simulink model "PID_Controller_Quadrotor"  (R2019b)
settings: Solver=VariableStepAuto  StartTime=0.0  StopTime=200  RelTol=1e-3
values from neighbouring files (symbols this model uses):
  b = 6.66e-5    (= 6.66e-05)    [LQR control.m]    (also in Parameters for PID.m)
  d = 1.642e-4    (= 0.0001642)    [Parameters for PID.m]
  g = 9.81    [Parameters for PID.m]
  Ixx = 155237782e-9    (= 0.155237782)    [LQR control.m]    (also in Parameters for PID.m)
  Iyy = 183039510e-9    (= 0.18303951)    [LQR control.m]    (also in Parameters for PID.m)
  Izz = 66119823e-9    (= 0.066119823)    [LQR control.m]    (also in Parameters for PID.m)
  Jr = 824e-6    (= 0.000824)    [Parameters for PID.m]
  l = 0.34    [Parameters for PID.m]
  m = 4    [LQR control.m]    (also in Parameters for PID.m)
undefined symbols (not defined in the file or in its folder): sigbuilder_block
libraries: simulink x4
settings Model: Creator=Dell  LastModifiedBy=Dell

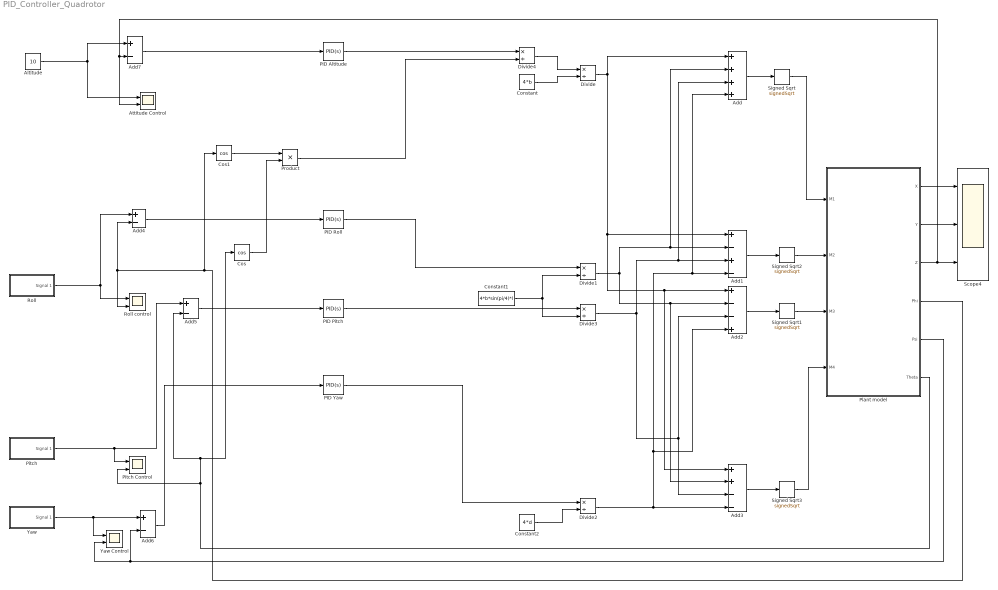
== system PID_Controller_Quadrotor ==
  " PID Altitude" : simulink/Continuous/PID Controller  Controller=PID  Form=Parallel  TimeDomain=Continuous-time  SampleTime=-1  IntegratorMethod=Forward Euler  FilterMethod=Forward Euler  ControllerParametersSource=internal  P=10  I=1.5  D=4.7  UseFilter=on  N=100  TunerSelectOption=Transfer Function Based (PID Tuner App)  InitialConditionSource=internal  InitialConditionForIntegrator=0  InitialConditionForFilter=0  DifferentiatorICPrevScaledInput=0  ExternalReset=none  TrackingMode=off  Kt=1  LimitOutput=off  UpperSaturationLimit=inf  LowerSaturationLimit=-inf  LinearizeAsGain=off  AntiWindupMode=none  Kb=1  POutMin=[]  POutMax=[]  IOutMin=[]  IOutMax=[]  DOutMin=[]  DOutMax=[]  NOutMin=[]  NOutMax=[]  SumOutMin=[]  SumOutMax=[]  SaturationOutMin=[]  SaturationOutMax=[]  PParamMin=[]  PParamMax=[]  IParamMin=[]  IParamMax=[]  DParamMin=[]  DParamMax=[]  NParamMin=[]  NParamMax=[]  KbParamMin=[]  KbParamMax=[]  KtParamMin=[]  KtParamMax=[]  KbOutMin=[]  KbOutMax=[]  KtOutMin=[]  KtOutMax=[]  IntegratorOutMin=[]  IntegratorOutMax=[]  FilterOutMin=[]  FilterOutMax=[]  SumI1OutMin=[]  SumI1OutMax=[]  SumI2OutMin=[]  SumI2OutMax=[]  SumI3OutMin=[]  SumI3OutMax=[]  SumI4OutMin=[]  SumI4OutMax=[]  SumDOutMin=[]  SumDOutMax=[]  DifferentiatorOutMin=[]  DifferentiatorOutMax=[]  FilterDiffOutCoefMin=[]  FilterDiffOutCoefMax=[]  ReciprocalOutMin=[]  ReciprocalOutMax=[]  SumDenOutMin=[]  SumDenOutMax=[]  SumNumOutMin=[]  SumNumOutMax=[]  DivideOutMin=[]  DivideOutMax=[]  IntegratorContinuousStateAttributes=''  IntegratorStateMustResolveToSignalObject=off  IntegratorRTWStateStorageClass=Auto  FilterContinuousStateAttributes=''  FilterStateMustResolveToSignalObject=off  FilterRTWStateStorageClass=Auto  ParallelPVariant=InternalParameters  IdealPVariant=Disabled  IVariant=InternalParameters  DVariant=InternalParameters  IntegratorVariant=Continuous  SatVariant=Disabled  AWVariant=Passthrough  PCopyVariant=Disabled  TRVariant=Disabled  FdbkBlocksVariant=Forward  IdealPFdbkVariant=Disabled  SatFdbkVariant=Disabled  DerivativeFilterVariant=ContFilter  NVariant=InternalParameters  NCopyVariant=Disabled  FilterICVariant=InternalICsFilter  IntegratorICVariant=InternalICs  ExternalResetVariant=Disabled  TRSumVariant=Passthrough  SumFdbkVariant=Disabled  SumVariant=Sum_PID
  " PID Pitch" : simulink/Continuous/PID Controller  Controller=PID  Form=Parallel  TimeDomain=Continuous-time  SampleTime=-1  IntegratorMethod=Forward Euler  FilterMethod=Forward Euler  ControllerParametersSource=internal  P=0.04  I=0  D=0.6  UseFilter=on  N=100  TunerSelectOption=Transfer Function Based (PID Tuner App)  InitialConditionSource=internal  InitialConditionForIntegrator=0  InitialConditionForFilter=0  DifferentiatorICPrevScaledInput=0  ExternalReset=none  TrackingMode=off  Kt=1  LimitOutput=off  UpperSaturationLimit=inf  LowerSaturationLimit=-inf  LinearizeAsGain=off  AntiWindupMode=none  Kb=1  POutMin=[]  POutMax=[]  IOutMin=[]  IOutMax=[]  DOutMin=[]  DOutMax=[]  NOutMin=[]  NOutMax=[]  SumOutMin=[]  SumOutMax=[]  SaturationOutMin=[]  SaturationOutMax=[]  PParamMin=[]  PParamMax=[]  IParamMin=[]  IParamMax=[]  DParamMin=[]  DParamMax=[]  NParamMin=[]  NParamMax=[]  KbParamMin=[]  KbParamMax=[]  KtParamMin=[]  KtParamMax=[]  KbOutMin=[]  KbOutMax=[]  KtOutMin=[]  KtOutMax=[]  IntegratorOutMin=[]  IntegratorOutMax=[]  FilterOutMin=[]  FilterOutMax=[]  SumI1OutMin=[]  SumI1OutMax=[]  SumI2OutMin=[]  SumI2OutMax=[]  SumI3OutMin=[]  SumI3OutMax=[]  SumI4OutMin=[]  SumI4OutMax=[]  SumDOutMin=[]  SumDOutMax=[]  DifferentiatorOutMin=[]  DifferentiatorOutMax=[]  FilterDiffOutCoefMin=[]  FilterDiffOutCoefMax=[]  ReciprocalOutMin=[]  ReciprocalOutMax=[]  SumDenOutMin=[]  SumDenOutMax=[]  SumNumOutMin=[]  SumNumOutMax=[]  DivideOutMin=[]  DivideOutMax=[]  IntegratorContinuousStateAttributes=''  IntegratorStateMustResolveToSignalObject=off  IntegratorRTWStateStorageClass=Auto  FilterContinuousStateAttributes=''  FilterStateMustResolveToSignalObject=off  FilterRTWStateStorageClass=Auto  ParallelPVariant=InternalParameters  IdealPVariant=Disabled  IVariant=InternalParameters  DVariant=InternalParameters  IntegratorVariant=Continuous  SatVariant=Disabled  AWVariant=Passthrough  PCopyVariant=Disabled  TRVariant=Disabled  FdbkBlocksVariant=Forward  IdealPFdbkVariant=Disabled  SatFdbkVariant=Disabled  DerivativeFilterVariant=ContFilter  NVariant=InternalParameters  NCopyVariant=Disabled  FilterICVariant=InternalICsFilter  IntegratorICVariant=InternalICs  ExternalResetVariant=Disabled  TRSumVariant=Passthrough  SumFdbkVariant=Disabled  SumVariant=Sum_PID
  " PID Roll" : simulink/Continuous/PID Controller  Controller=PID  Form=Parallel  TimeDomain=Continuous-time  SampleTime=-1  IntegratorMethod=Forward Euler  FilterMethod=Forward Euler  ControllerParametersSource=internal  P=0.001  I=0  D=0.13  UseFilter=on  N=100  TunerSelectOption=Transfer Function Based (PID Tuner App)  InitialConditionSource=internal  InitialConditionForIntegrator=0  InitialConditionForFilter=0  DifferentiatorICPrevScaledInput=0  ExternalReset=none  TrackingMode=off  Kt=1  LimitOutput=off  UpperSaturationLimit=inf  LowerSaturationLimit=-inf  LinearizeAsGain=off  AntiWindupMode=none  Kb=1  POutMin=[]  POutMax=[]  IOutMin=[]  IOutMax=[]  DOutMin=[]  DOutMax=[]  NOutMin=[]  NOutMax=[]  SumOutMin=[]  SumOutMax=[]  SaturationOutMin=[]  SaturationOutMax=[]  PParamMin=[]  PParamMax=[]  IParamMin=[]  IParamMax=[]  DParamMin=[]  DParamMax=[]  NParamMin=[]  NParamMax=[]  KbParamMin=[]  KbParamMax=[]  KtParamMin=[]  KtParamMax=[]  KbOutMin=[]  KbOutMax=[]  KtOutMin=[]  KtOutMax=[]  IntegratorOutMin=[]  IntegratorOutMax=[]  FilterOutMin=[]  FilterOutMax=[]  SumI1OutMin=[]  SumI1OutMax=[]  SumI2OutMin=[]  SumI2OutMax=[]  SumI3OutMin=[]  SumI3OutMax=[]  SumI4OutMin=[]  SumI4OutMax=[]  SumDOutMin=[]  SumDOutMax=[]  DifferentiatorOutMin=[]  DifferentiatorOutMax=[]  FilterDiffOutCoefMin=[]  FilterDiffOutCoefMax=[]  ReciprocalOutMin=[]  ReciprocalOutMax=[]  SumDenOutMin=[]  SumDenOutMax=[]  SumNumOutMin=[]  SumNumOutMax=[]  DivideOutMin=[]  DivideOutMax=[]  IntegratorContinuousStateAttributes=''  IntegratorStateMustResolveToSignalObject=off  IntegratorRTWStateStorageClass=Auto  FilterContinuousStateAttributes=''  FilterStateMustResolveToSignalObject=off  FilterRTWStateStorageClass=Auto  ParallelPVariant=InternalParameters  IdealPVariant=Disabled  IVariant=InternalParameters  DVariant=InternalParameters  IntegratorVariant=Continuous  SatVariant=Disabled  AWVariant=Passthrough  PCopyVariant=Disabled  TRVariant=Disabled  FdbkBlocksVariant=Forward  IdealPFdbkVariant=Disabled  SatFdbkVariant=Disabled  DerivativeFilterVariant=ContFilter  NVariant=InternalParameters  NCopyVariant=Disabled  FilterICVariant=InternalICsFilter  IntegratorICVariant=InternalICs  ExternalResetVariant=Disabled  TRSumVariant=Passthrough  SumFdbkVariant=Disabled  SumVariant=Sum_PID
  " PID Yaw" : simulink/Continuous/PID Controller  Controller=PID  Form=Parallel  TimeDomain=Continuous-time  SampleTime=-1  IntegratorMethod=Forward Euler  FilterMethod=Forward Euler  ControllerParametersSource=internal  P=0.001  I=0  D=0.6  UseFilter=on  N=100  TunerSelectOption=Transfer Function Based (PID Tuner App)  InitialConditionSource=internal  InitialConditionForIntegrator=0  InitialConditionForFilter=0  DifferentiatorICPrevScaledInput=0  ExternalReset=none  TrackingMode=off  Kt=1  LimitOutput=off  UpperSaturationLimit=inf  LowerSaturationLimit=-inf  LinearizeAsGain=off  AntiWindupMode=none  Kb=1  POutMin=[]  POutMax=[]  IOutMin=[]  IOutMax=[]  DOutMin=[]  DOutMax=[]  NOutMin=[]  NOutMax=[]  SumOutMin=[]  SumOutMax=[]  SaturationOutMin=[]  SaturationOutMax=[]  PParamMin=[]  PParamMax=[]  IParamMin=[]  IParamMax=[]  DParamMin=[]  DParamMax=[]  NParamMin=[]  NParamMax=[]  KbParamMin=[]  KbParamMax=[]  KtParamMin=[]  KtParamMax=[]  KbOutMin=[]  KbOutMax=[]  KtOutMin=[]  KtOutMax=[]  IntegratorOutMin=[]  IntegratorOutMax=[]  FilterOutMin=[]  FilterOutMax=[]  SumI1OutMin=[]  SumI1OutMax=[]  SumI2OutMin=[]  SumI2OutMax=[]  SumI3OutMin=[]  SumI3OutMax=[]  SumI4OutMin=[]  SumI4OutMax=[]  SumDOutMin=[]  SumDOutMax=[]  DifferentiatorOutMin=[]  DifferentiatorOutMax=[]  FilterDiffOutCoefMin=[]  FilterDiffOutCoefMax=[]  ReciprocalOutMin=[]  ReciprocalOutMax=[]  SumDenOutMin=[]  SumDenOutMax=[]  SumNumOutMin=[]  SumNumOutMax=[]  DivideOutMin=[]  DivideOutMax=[]  IntegratorContinuousStateAttributes=''  IntegratorStateMustResolveToSignalObject=off  IntegratorRTWStateStorageClass=Auto  FilterContinuousStateAttributes=''  FilterStateMustResolveToSignalObject=off  FilterRTWStateStorageClass=Auto  ParallelPVariant=InternalParameters  IdealPVariant=Disabled  IVariant=InternalParameters  DVariant=InternalParameters  IntegratorVariant=Continuous  SatVariant=Disabled  AWVariant=Passthrough  PCopyVariant=Disabled  TRVariant=Disabled  FdbkBlocksVariant=Forward  IdealPFdbkVariant=Disabled  SatFdbkVariant=Disabled  DerivativeFilterVariant=ContFilter  NVariant=InternalParameters  NCopyVariant=Disabled  FilterICVariant=InternalICsFilter  IntegratorICVariant=InternalICs  ExternalResetVariant=Disabled  TRSumVariant=Passthrough  SumFdbkVariant=Disabled  SumVariant=Sum_PID
  Add : Sum  Inputs=++++
  Add1 : Sum  Inputs=+-+-
  Add2 : Sum  Inputs=+--+
  Add3 : Sum  Inputs=++--
  Add{4..7} (4 alike) : Sum  Inputs=+-
  "Altitude " : Constant  Value=10
  "Attitude Control " : Scope  NumInputPorts=2
  Constant : Constant  Value=4*b
  Constant1 : Constant  Value=4*b*sin(pi/4)*l
  Constant2 : Constant  Value=4*d
  Cos : Trigonometry  Operator=cos
  Cos1 : Trigonometry  Operator=cos
  Divide{,1..4} (5 alike) : Product  Inputs=*/
  Pitch : Subsystem  Tag=STV Subsys  LoadFcn=sigbuilder_block('load');  StartFcn=sigbuilder_block('start');  StopFcn=sigbuilder_block('stop');  ClipboardFcn=sigbuilder_block('clipboard');  mask(Sigbuilder block){tuvar=[0:10]}
      mask help: Simulink:masks:SigbuilderBlock_MD
      mask init:
      | if ~strcmp(get_param(bdroot(gcbh),'SimulationStatus'),'stopped') tuvar = sigbuilder_block('maskInit'); end
      settings: CopyFcn=sigbuilder_block('copy');  DeleteFcn=sigbuilder_block('delete');  ModelCloseFcn=sigbuilder_block('modelClose');  PreSaveFcn=sigbuilder_block('preSave');  PauseFcn=sigbuilder_block('pause');  ContinueFcn=sigbuilder_block('continue');  NameChangeFcn=sigbuilder_block('namechange');  OpenFcn=sigbuilder_block('open',[437.6 199.2 550.4 400 ]);  CloseFcn=sigbuilder_block('close');
      mask Display: plot(0, 0, 100, 100,[2, 2, 32, 32, 2], [68, 8, 8, 68, 68],[32, 2], [38, 38], [32, 19, 2],[53, 60, 44], [32, 17, 17, 2],[16, 16, 31, 31]);txt = getActiveGroup(gcbh);text(2, 100, txt,'verticalAlignment', 'top');
  Pitch Control : Scope  NumInputPorts=2
  "Plant model " : Subsystem
  Product : Product
  Roll : Subsystem  Tag=STV Subsys  LoadFcn=sigbuilder_block('load');  StartFcn=sigbuilder_block('start');  StopFcn=sigbuilder_block('stop');  ClipboardFcn=sigbuilder_block('clipboard');  mask(Sigbuilder block){tuvar=[0:10]}
      mask help: Simulink:masks:SigbuilderBlock_MD
      mask init:
      | if ~strcmp(get_param(bdroot(gcbh),'SimulationStatus'),'stopped') tuvar = sigbuilder_block('maskInit'); end
      settings: CopyFcn=sigbuilder_block('copy');  DeleteFcn=sigbuilder_block('delete');  ModelCloseFcn=sigbuilder_block('modelClose');  PreSaveFcn=sigbuilder_block('preSave');  PauseFcn=sigbuilder_block('pause');  ContinueFcn=sigbuilder_block('continue');  NameChangeFcn=sigbuilder_block('namechange');  OpenFcn=sigbuilder_block('open',[437.6 199.2 550.4 400 ]);  CloseFcn=sigbuilder_block('close');
      mask Display: plot(0, 0, 100, 100,[2, 2, 32, 32, 2], [68, 8, 8, 68, 68],[32, 2], [38, 38], [32, 19, 2],[53, 60, 44], [32, 17, 17, 2],[16, 16, 31, 31]);txt = getActiveGroup(gcbh);text(2, 100, txt,'verticalAlignment', 'top');
  Roll control : Scope  NumInputPorts=2
  Scope4 : Scope  NumInputPorts=3
  Signed Sqrt{,1..3} (4 alike) : Sqrt  Operator=signedSqrt  SaturateOnIntegerOverflow=on
  Yaw : Subsystem  Tag=STV Subsys  LoadFcn=sigbuilder_block('load');  StartFcn=sigbuilder_block('start');  StopFcn=sigbuilder_block('stop');  ClipboardFcn=sigbuilder_block('clipboard');  mask(Sigbuilder block){tuvar=[0:10]}
      mask help: Simulink:masks:SigbuilderBlock_MD
      mask init:
      | if ~strcmp(get_param(bdroot(gcbh),'SimulationStatus'),'stopped') tuvar = sigbuilder_block('maskInit'); end
      settings: CopyFcn=sigbuilder_block('copy');  DeleteFcn=sigbuilder_block('delete');  ModelCloseFcn=sigbuilder_block('modelClose');  PreSaveFcn=sigbuilder_block('preSave');  PauseFcn=sigbuilder_block('pause');  ContinueFcn=sigbuilder_block('continue');  NameChangeFcn=sigbuilder_block('namechange');  OpenFcn=sigbuilder_block('open',[437.6 199.2 550.4 400 ]);  CloseFcn=sigbuilder_block('close');
      mask Display: plot(0, 0, 100, 100,[2, 2, 32, 32, 2], [68, 8, 8, 68, 68],[32, 2], [38, 38], [32, 19, 2],[53, 60, 44], [32, 17, 17, 2],[16, 16, 31, 31]);txt = getActiveGroup(gcbh);text(2, 100, txt,'verticalAlignment', 'top');
  Yaw Control : Scope  NumInputPorts=2
  wires:
  Add1/1 -> Signed Sqrt2/1
  Add/1 -> Signed Sqrt/1
  Add2/1 -> Signed Sqrt1/1
  Add3/1 -> Signed Sqrt3/1
  Signed Sqrt/1 -> "Plant model "/1(M1)
  Signed Sqrt2/1 -> "Plant model "/2(M2)
  Signed Sqrt1/1 -> "Plant model "/3(M3)
  Signed Sqrt3/1 -> "Plant model "/4(M4)
  Divide/1 -> Add/1, Add3/1, Add2/1, Add1/1
  Divide1/1 -> Add1/2, Add/2, Add3/2, Add2/2
  Divide3/1 -> Add1/3, Add/3, Add3/3, Add2/3
  Divide2/1 -> Add3/4, Add2/4, Add/4, Add1/4
  Constant1/1 -> Divide1/2, Divide3/2
  Constant/1 -> Divide/2
  Constant2/1 -> Divide2/2
  Roll/1(Signal 1) -> Add4/1, Roll control/1
  Yaw/1(Signal 1) -> Yaw Control/1, Add6/1
  Pitch/1(Signal 1) -> Pitch Control/1, Add5/1
  "Plant model "/6(Theta) -> Pitch Control/2, Cos/1, Add5/2
  Cos1/1 -> Product/1
  "Plant model "/5("Psi ") -> Yaw Control/2, Add6/2
  "Plant model "/4(Phi) -> Cos1/1, Add4/2, Roll control/2
  Cos/1 -> Product/2
  Product/1 -> Divide4/2
  "Plant model "/3(Z) -> Scope4/3, "Attitude Control "/2, Add7/2
  "Altitude "/1 -> "Attitude Control "/1, Add7/1
  "Plant model "/1(X) -> Scope4/1
  "Plant model "/2(Y) -> Scope4/2
  Divide4/1 -> Divide/1
  " PID Altitude"/1 -> Divide4/1
  " PID Roll"/1 -> Divide1/1
  " PID Pitch"/1 -> Divide3/1
  " PID Yaw"/1 -> Divide2/1
  Add6/1 -> " PID Yaw"/1
  Add4/1 -> " PID Roll"/1
  Add5/1 -> " PID Pitch"/1
  Add7/1 -> " PID Altitude"/1

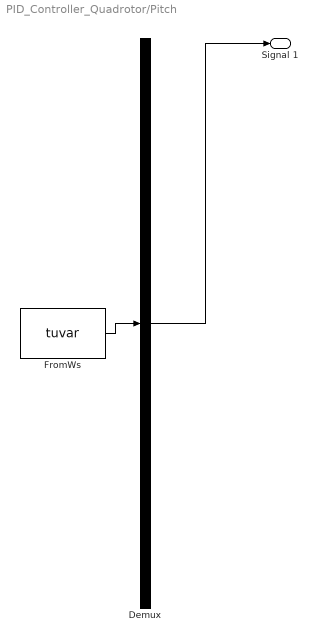
== system PID_Controller_Quadrotor/Pitch ==
  Demux : Demux  Tag=STV Demux  Outputs=1
  FromWs : FromWorkspace  Tag=STV FromWs  VariableName=tuvar  SampleTime=0
      SigBuilderData=|
      | common.afterFinalStr = 'Extrapolate'
      | common.sampleTime = 0
      | dataSet.timeRange = [0 1000]
      | dataSet.name = 'Group 1'
      | sbobj.Groups.Name = 'Group 1'
      | sbobj.Groups.Signals.Name = 'Signal 1'
      | sbobj.Groups.Signals.XData = [0 80 80 110 110 1000]
      | sbobj.Groups.Signals.YData = [0 0 0.2 0.2 0 0]
      | sbobj.Groups.TimeRange = [0 1000]
  Signal 1 : Outport  Tag=STV Outport
  wires:
  Demux/1 -> Signal 1/1
  FromWs/1 -> Demux/1

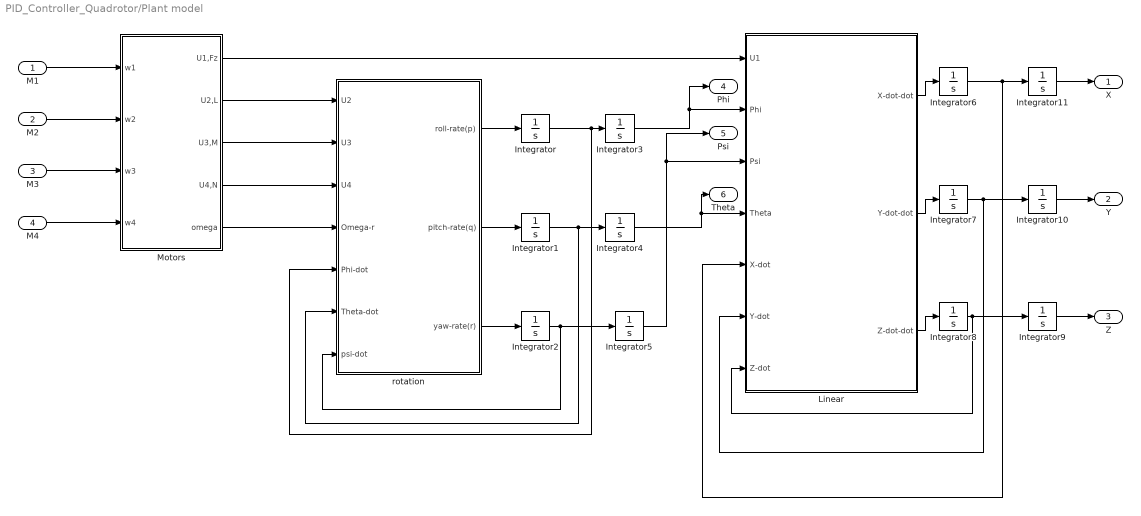
== system PID_Controller_Quadrotor/Plant model  ==
  M1 : Inport
  M2 : Inport  Port=2
  M3 : Inport  Port=3
  M4 : Inport  Port=4
  Integrator{,1..2,6..8} (6 alike) : Integrator
  Integrator10 : Integrator  LimitOutput=on
  Integrator11 : Integrator  LimitOutput=on
  Integrator3 : Integrator  WrapState=on
  Integrator4 : Integrator  WrapState=on
  Integrator5 : Integrator  WrapState=on
  Integrator9 : Integrator  LimitOutput=on
  "Linear " : Subsystem
  Motors : Subsystem
  "rotation " : Subsystem
  X : Outport
  Y : Outport  Port=2
  Z : Outport  Port=3
  Phi : Outport  Port=4
  "Psi " : Outport  Port=5
  Theta : Outport  Port=6
  wires:
  Integrator8/1 -> "Linear "/7("Z-dot "), Integrator9/1
  Motors/5("omega ") -> "rotation "/4("Omega-r ")
  Motors/4(U4,N) -> "rotation "/3(U4)
  Integrator2/1 -> Integrator5/1, "rotation "/7("psi-dot ")
  Integrator7/1 -> "Linear "/6(Y-dot), Integrator10/1
  M4/1 -> Motors/4(w4)
  "Linear "/1(X-dot-dot) -> Integrator6/1
  Integrator6/1 -> "Linear "/5("X-dot "), Integrator11/1
  Integrator5/1 -> "Psi "/1, "Linear "/3("Psi ")
  "rotation "/3(yaw-rate(r)) -> Integrator2/1
  M3/1 -> Motors/3(w3)
  "Linear "/2(Y-dot-dot) -> Integrator7/1
  Integrator3/1 -> "Linear "/2(Phi), Phi/1
  Motors/3("U3,M ") -> "rotation "/2(U3)
  Integrator9/1 -> Z/1
  Integrator1/1 -> "rotation "/6("Theta-dot "), Integrator4/1
  Integrator/1 -> "rotation "/5("Phi-dot "), Integrator3/1
  Integrator4/1 -> Theta/1, "Linear "/4(Theta)
  Motors/2(U2,L) -> "rotation "/1(U2)
  Integrator11/1 -> X/1
  Integrator10/1 -> Y/1
  M2/1 -> Motors/2(w2)
  "rotation "/2(pitch-rate(q)) -> Integrator1/1
  M1/1 -> Motors/1(w1)
  "Linear "/3(Z-dot-dot) -> Integrator8/1
  "rotation "/1(roll-rate(p)) -> Integrator/1
  Motors/1("U1,Fz ") -> "Linear "/1(U1)

== system PID_Controller_Quadrotor/Roll ==
  Demux : Demux  Tag=STV Demux  Outputs=1
  FromWs : FromWorkspace  Tag=STV FromWs  VariableName=tuvar  SampleTime=0
      SigBuilderData=|
      | common.afterFinalStr = 'Extrapolate'
      | common.sampleTime = 0
      | dataSet.timeRange = [0 1000]
      | dataSet.name = 'Group 1'
      | sbobj.Groups.Name = 'Group 1'
      | sbobj.Groups.Signals.Name = 'Signal 1'
      | sbobj.Groups.Signals.XData = [0 10 10 60 60 1000]
      | sbobj.Groups.Signals.YData = [0 0 0.2 0.2 0 0]
      | sbobj.Groups.TimeRange = [0 1000]
  Signal 1 : Outport  Tag=STV Outport
  wires:
  Demux/1 -> Signal 1/1
  FromWs/1 -> Demux/1

== system PID_Controller_Quadrotor/Yaw ==
  Demux : Demux  Tag=STV Demux  Outputs=1
  FromWs : FromWorkspace  Tag=STV FromWs  VariableName=tuvar  SampleTime=0
      SigBuilderData=|
      | common.afterFinalStr = 'Extrapolate'
      | common.sampleTime = 0
      | dataSet.timeRange = [0 1000]
      | dataSet.name = 'Group 1'
      | sbobj.Groups.Name = 'Group 1'
      | sbobj.Groups.Signals.Name = 'Signal 1'
      | sbobj.Groups.Signals.XData = [0 120 120 150 150 1000]
      | sbobj.Groups.Signals.YData = [0 0 0.2 0.2 0 0]
      | sbobj.Groups.TimeRange = [0 1000]
  Signal 1 : Outport  Tag=STV Outport
  wires:
  Demux/1 -> Signal 1/1
  FromWs/1 -> Demux/1

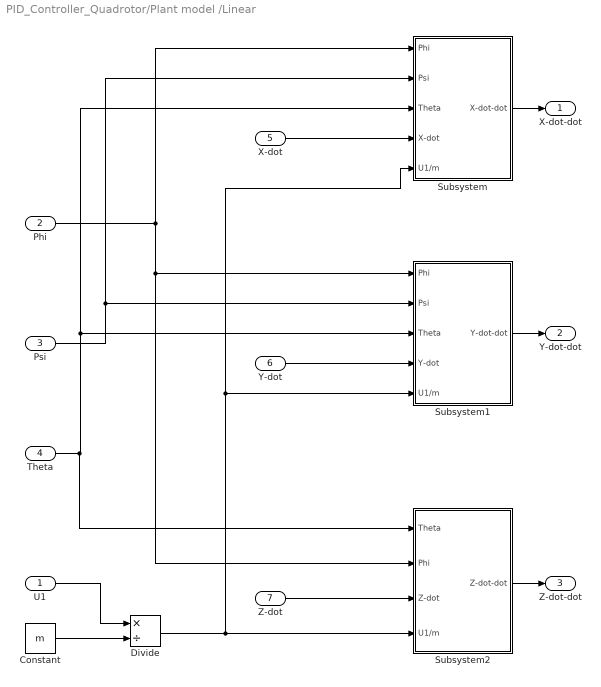
== system PID_Controller_Quadrotor/Plant model /Linear  ==
  U1 : Inport
  Phi : Inport  Port=2
  "Psi " : Inport  Port=3
  Theta : Inport  Port=4
  "X-dot " : Inport  Port=5
  Y-dot : Inport  Port=6
  "Z-dot " : Inport  Port=7
  Constant : Constant  Value=m
  Divide : Product  Inputs=*/
  Subsystem : Subsystem
  Subsystem1 : Subsystem
  Subsystem2 : Subsystem
  X-dot-dot : Outport
  Y-dot-dot : Outport  Port=2
  Z-dot-dot : Outport  Port=3
  wires:
  Phi/1 -> Subsystem/1(Phi), Subsystem2/2(Phi), Subsystem1/1(Phi)
  "Psi "/1 -> Subsystem1/2("Psi "), Subsystem/2("Psi ")
  Theta/1 -> Subsystem2/1(Theta), Subsystem1/3(Theta), Subsystem/3(Theta)
  "X-dot "/1 -> Subsystem/4("X-dot ")
  Subsystem/1(X-dot-dot) -> X-dot-dot/1
  U1/1 -> Divide/1
  Constant/1 -> Divide/2
  Divide/1 -> Subsystem1/5(U1/m), Subsystem/5(U1/m), Subsystem2/4(U1/m)
  Y-dot/1 -> Subsystem1/4("Y-dot ")
  "Z-dot "/1 -> Subsystem2/3("Z-dot ")
  Subsystem2/1(Z-dot-dot) -> Z-dot-dot/1
  Subsystem1/1(Y-dot-dot) -> Y-dot-dot/1

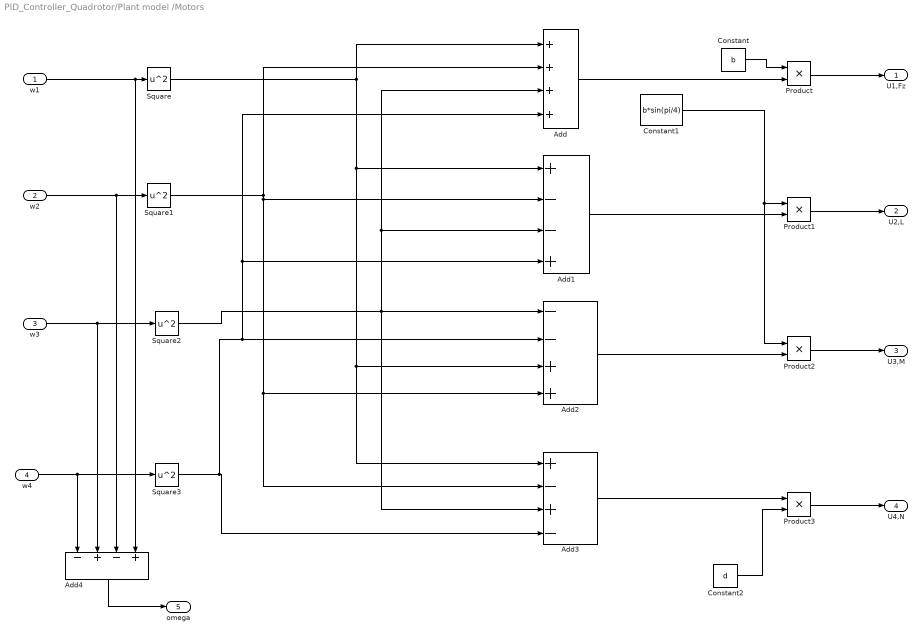
== system PID_Controller_Quadrotor/Plant model /Motors ==
  w1 : Inport
  w2 : Inport  Port=2
  w3 : Inport  Port=3
  w4 : Inport  Port=4
  Add : Sum  Inputs=++++
  Add1 : Sum  Inputs=+--+
  Add2 : Sum  Inputs=--++
  Add3 : Sum  Inputs=+-+-
  Add4 : Sum  Inputs=-+-+
  Constant : Constant  Value=b
  Constant1 : Constant  Value=b*sin(pi/4)
  Constant2 : Constant  Value=d
  Product{,1..3} (4 alike) : Product
  Square{,1..3} (4 alike) : Math  Operator=square  SignedPower=off  SaturateOnIntegerOverflow=on
  "U1,Fz " : Outport
  U2,L : Outport  Port=2
  "U3,M " : Outport  Port=3
  U4,N : Outport  Port=4
  "omega " : Outport  Port=5
  wires:
  Product/1 -> "U1,Fz "/1
  Constant2/1 -> Product3/2
  Product2/1 -> "U3,M "/1
  w2/1 -> Square1/1, Add4/3
  Constant1/1 -> Product2/1, Product1/1
  w1/1 -> Add4/4, Square/1
  Square/1 -> Add3/1, Add2/3, Add1/1, Add/1
  Add1/1 -> Product1/2
  w3/1 -> Square2/1, Add4/2
  Square1/1 -> Add/2, Add3/2, Add2/4, Add1/2
  Square2/1 -> Add3/3, Add1/3, Add/3, Add2/1
  Square3/1 -> Add/4, Add1/4, Add2/2, Add3/4
  Product3/1 -> U4,N/1
  Add3/1 -> Product3/1
  Add4/1 -> "omega "/1
  Add/1 -> Product/2
  Constant/1 -> Product/1
  w4/1 -> Square3/1, Add4/1
  Add2/1 -> Product2/2
  Product1/1 -> U2,L/1

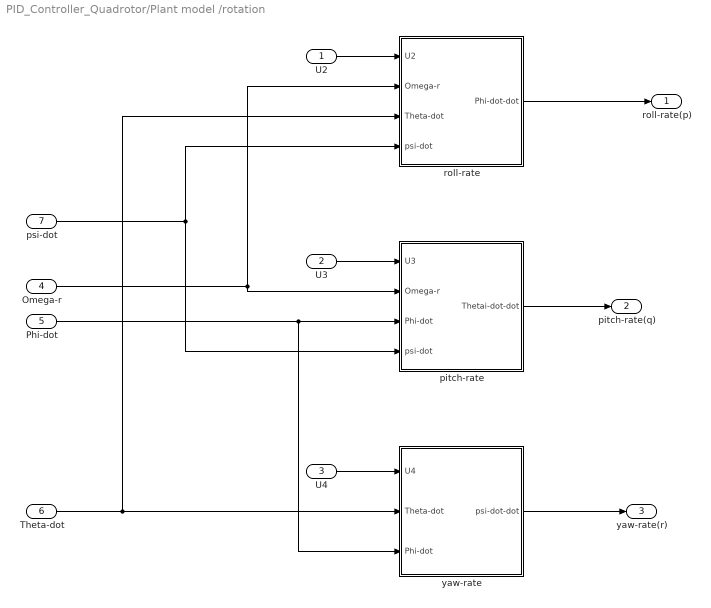
== system PID_Controller_Quadrotor/Plant model /rotation  ==
  U2 : Inport
  U3 : Inport  Port=2
  U4 : Inport  Port=3
  "Omega-r " : Inport  Port=4
  "Phi-dot " : Inport  Port=5
  "Theta-dot " : Inport  Port=6
  "psi-dot " : Inport  Port=7
  pitch-rate : Subsystem
  "roll-rate " : Subsystem
  yaw-rate : Subsystem
  roll-rate(p) : Outport
  pitch-rate(q) : Outport  Port=2
  yaw-rate(r) : Outport  Port=3
  wires:
  U2/1 -> "roll-rate "/1(U2)
  "Omega-r "/1 -> pitch-rate/2("Omega-r "), "roll-rate "/2("Omega-r ")
  "Theta-dot "/1 -> "roll-rate "/3("Theta-dot "), yaw-rate/2("Theta-dot ")
  "psi-dot "/1 -> "roll-rate "/4("psi-dot "), pitch-rate/4("psi-dot ")
  "roll-rate "/1(Phi-dot-dot) -> roll-rate(p)/1
  U3/1 -> pitch-rate/1(U3)
  U4/1 -> yaw-rate/1(U4)
  "Phi-dot "/1 -> yaw-rate/3("Phi-dot "), pitch-rate/3("Phi-dot ")
  yaw-rate/1(psi-dot-dot) -> yaw-rate(r)/1
  pitch-rate/1(Thetai-dot-dot) -> pitch-rate(q)/1

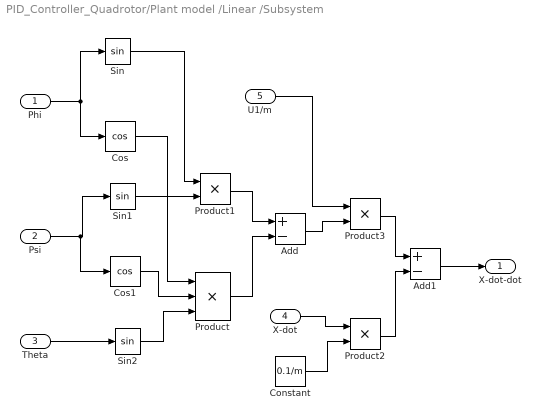
== system PID_Controller_Quadrotor/Plant model /Linear /Subsystem ==
  Phi : Inport
  "Psi " : Inport  Port=2
  Theta : Inport  Port=3
  "X-dot " : Inport  Port=4
  U1/m : Inport  Port=5
  Add : Sum  Inputs=+-
  Add1 : Sum  Inputs=+-
  Constant : Constant  Value=0.1/m
  Cos : Trigonometry  Operator=cos
  Cos1 : Trigonometry  Operator=cos
  Product : Product  Inputs=3
  Product1 : Product
  Product2 : Product
  Product3 : Product
  Sin : Trigonometry
  Sin1 : Trigonometry
  Sin2 : Trigonometry
  X-dot-dot : Outport
  wires:
  U1/m/1 -> Product3/1
  Phi/1 -> Cos/1, Sin/1
  Constant/1 -> Product2/2
  Sin/1 -> Product1/1
  Product2/1 -> Add1/2
  Add/1 -> Product3/2
  "Psi "/1 -> Cos1/1, Sin1/1
  Sin1/1 -> Product1/2
  Cos/1 -> Product/1
  "X-dot "/1 -> Product2/1
  Cos1/1 -> Product/2
  Product1/1 -> Add/1
  Product/1 -> Add/2
  Product3/1 -> Add1/1
  Sin2/1 -> Product/3
  Theta/1 -> Sin2/1
  Add1/1 -> X-dot-dot/1

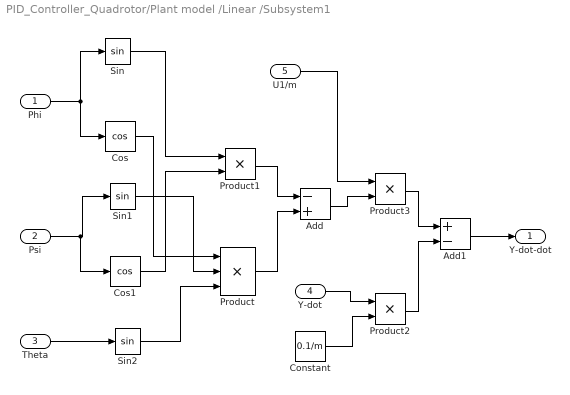
== system PID_Controller_Quadrotor/Plant model /Linear /Subsystem1 ==
  Phi : Inport
  "Psi " : Inport  Port=2
  Theta : Inport  Port=3
  "Y-dot " : Inport  Port=4
  U1/m : Inport  Port=5
  Add : Sum  Inputs=-+
  Add1 : Sum  Inputs=+-
  Constant : Constant  Value=0.1/m
  Cos : Trigonometry  Operator=cos
  Cos1 : Trigonometry  Operator=cos
  Product : Product  Inputs=3
  Product1 : Product
  Product2 : Product
  Product3 : Product
  Sin : Trigonometry
  Sin1 : Trigonometry
  Sin2 : Trigonometry
  Y-dot-dot : Outport
  wires:
  U1/m/1 -> Product3/1
  Phi/1 -> Cos/1, Sin/1
  Constant/1 -> Product2/2
  Sin/1 -> Product1/1
  Product2/1 -> Add1/2
  Add/1 -> Product3/2
  "Psi "/1 -> Cos1/1, Sin1/1
  Cos/1 -> Product/1
  "Y-dot "/1 -> Product2/1
  Product1/1 -> Add/1
  Product/1 -> Add/2
  Product3/1 -> Add1/1
  Sin2/1 -> Product/3
  Theta/1 -> Sin2/1
  Add1/1 -> Y-dot-dot/1
  Cos1/1 -> Product1/2
  Sin1/1 -> Product/2

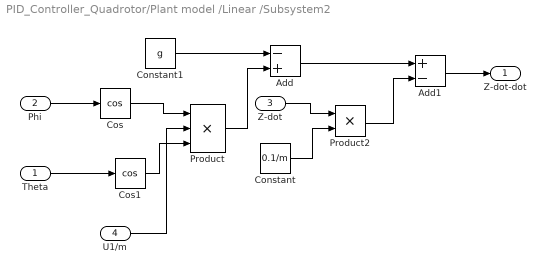
== system PID_Controller_Quadrotor/Plant model /Linear /Subsystem2 ==
  Theta : Inport
  Phi : Inport  Port=2
  "Z-dot " : Inport  Port=3
  U1/m : Inport  Port=4
  Add : Sum  Inputs=-+
  Add1 : Sum  Inputs=+-
  Constant : Constant  Value=0.1/m
  Constant1 : Constant  Value=g
  Cos : Trigonometry  Operator=cos
  Cos1 : Trigonometry  Operator=cos
  Product : Product  Inputs=3
  Product2 : Product
  Z-dot-dot : Outport
  wires:
  Constant/1 -> Product2/2
  Product2/1 -> Add1/2
  Phi/1 -> Cos/1
  "Z-dot "/1 -> Product2/1
  Constant1/1 -> Add/1
  Product/1 -> Add/2
  Add/1 -> Add1/1
  Cos1/1 -> Product/3
  Theta/1 -> Cos1/1
  Add1/1 -> Z-dot-dot/1
  Cos/1 -> Product/1
  U1/m/1 -> Product/2

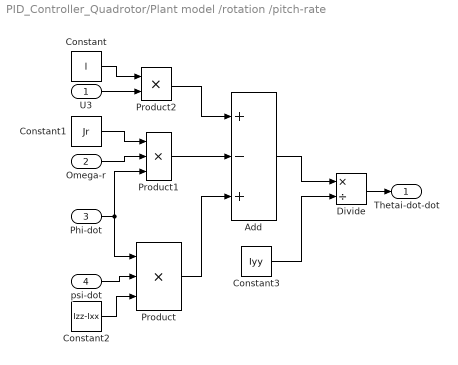
== system PID_Controller_Quadrotor/Plant model /rotation /pitch-rate ==
  U3 : Inport
  "Omega-r " : Inport  Port=2
  "Phi-dot " : Inport  Port=3
  "psi-dot " : Inport  Port=4
  Add : Sum  Inputs=+-+
  Constant : Constant  Value=l
  Constant1 : Constant  Value=Jr
  Constant2 : Constant  Value=Izz-Ixx
  Constant3 : Constant  Value=Iyy
  Divide : Product  Inputs=*/
  Product : Product  Inputs=3
  Product1 : Product  Inputs=3
  Product2 : Product
  Thetai-dot-dot : Outport
  wires:
  "psi-dot "/1 -> Product/2
  Constant1/1 -> Product1/1
  "Omega-r "/1 -> Product1/2
  "Phi-dot "/1 -> Product/1, Product1/3
  Constant/1 -> Product2/1
  U3/1 -> Product2/2
  Add/1 -> Divide/1
  Product2/1 -> Add/1
  Product1/1 -> Add/2
  Product/1 -> Add/3
  Constant2/1 -> Product/3
  Divide/1 -> Thetai-dot-dot/1
  Constant3/1 -> Divide/2

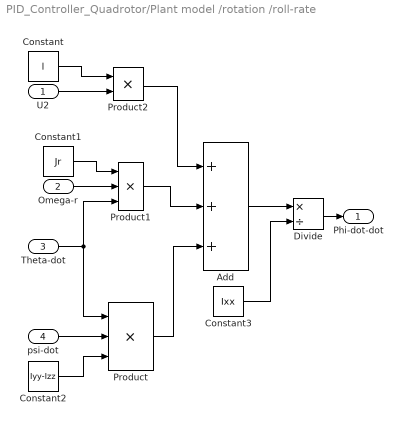
== system PID_Controller_Quadrotor/Plant model /rotation /roll-rate  ==
  U2 : Inport
  "Omega-r " : Inport  Port=2
  "Theta-dot " : Inport  Port=3
  "psi-dot " : Inport  Port=4
  Add : Sum  Inputs=+++
  Constant : Constant  Value=l
  Constant1 : Constant  Value=Jr
  Constant2 : Constant  Value=Iyy-Izz
  Constant3 : Constant  Value=Ixx
  Divide : Product  Inputs=*/
  Product : Product  Inputs=3
  Product1 : Product  Inputs=3
  Product2 : Product
  Phi-dot-dot : Outport
  wires:
  "psi-dot "/1 -> Product/2
  Constant1/1 -> Product1/1
  "Omega-r "/1 -> Product1/2
  "Theta-dot "/1 -> Product/1, Product1/3
  Constant/1 -> Product2/1
  U2/1 -> Product2/2
  Add/1 -> Divide/1
  Product2/1 -> Add/1
  Product1/1 -> Add/2
  Product/1 -> Add/3
  Constant2/1 -> Product/3
  Divide/1 -> Phi-dot-dot/1
  Constant3/1 -> Divide/2

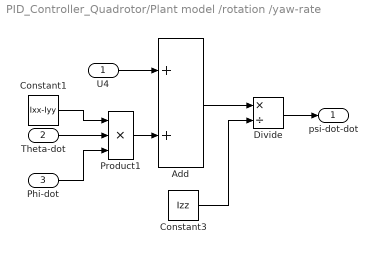
== system PID_Controller_Quadrotor/Plant model /rotation /yaw-rate ==
  U4 : Inport
  "Theta-dot " : Inport  Port=2
  "Phi-dot " : Inport  Port=3
  Add : Sum
  Constant1 : Constant  Value=Ixx-Iyy
  Constant3 : Constant  Value=Izz
  Divide : Product  Inputs=*/
  Product1 : Product  Inputs=3
  psi-dot-dot : Outport
  wires:
  Constant1/1 -> Product1/1
  "Theta-dot "/1 -> Product1/2
  "Phi-dot "/1 -> Product1/3
  Add/1 -> Divide/1
  Product1/1 -> Add/2
  Divide/1 -> psi-dot-dot/1
  Constant3/1 -> Divide/2
  U4/1 -> Add/1
